simulink model "Final_hand_model"  (R2020b)
settings: Solver=VariableStepAuto  StartTime=0.0  StopTime=10.0  RelTol=1e-3  AbsTol=1e-3  EnableMultiTasking=on
values from neighbouring files (symbols this model uses):
  Out = 0    [Gesture_code_to_use_network_Arduino.m]    (also in Gesture_code_to_use_network_Both.m; Gesture_code_to_use_network_Simulink.m)
undefined symbols (not defined in the file or in its folder): X, Y, Z
libraries: sm_lib x78, nesl_utility x16
(part 1 of 3)
settings Model: Creator=Joshu  LastModifiedBy=Joshu
settings SolverCC: AutoScaleAbsTol=off
settings DataIOCC: LimitDataPoints=on  MaxDataPoints=10000
settings OptimizationCC: LifeSpan=inf
settings DebuggingCC: AllowSymbolicDim=off  SFUnexpectedBacktrackingDiag=warning  SFNoUnconditionalDefaultTransitionDiag=warning  SFExecutionAtInitializationDiag=none  ArithmeticOperatorsInVariantConditions=warning
settings SFSimCC: SimUseLocalCustomCode=off  CustomCodeUndefinedFunction=UseInterfaceOnly
settings RTWCC: RTWUseLocalCustomCode=off
settings CodeAppCC: StateflowObjectComments=on
settings GRTTargetCC: TargetLangStandard=C89/C90 (ANSI)
settings ConfigComp: CovMetricSettings=dw  CovSaveCumulativeToWorkspaceVar=on  CovSaveSingleToWorkspaceVar=on  CovExternalEMLEnable=off  CovSFcnEnable=off
settings SimscapeCC: SimscapeLogType=all  SimscapeLogSimulationStatistics=on  SimscapeLogDataHistory=10000

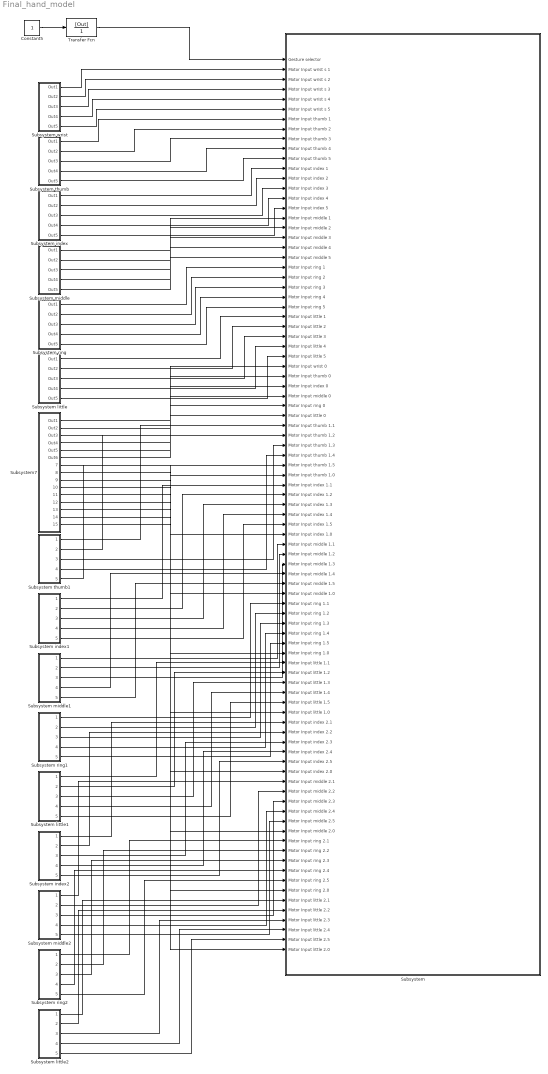
== system Final_hand_model ==
  Constant5 : Constant
  Subsystem : Subsystem
  Subsystem index : Subsystem
  Subsystem index1 : Subsystem
  Subsystem index2 : Subsystem
  Subsystem little : Subsystem
  Subsystem little1 : Subsystem
  Subsystem little2 : Subsystem
  Subsystem middle : Subsystem
  Subsystem middle1 : Subsystem
  Subsystem middle2 : Subsystem
  Subsystem ring : Subsystem
  Subsystem ring1 : Subsystem
  Subsystem ring2 : Subsystem
  Subsystem thumb : Subsystem
  Subsystem thumb1 : Subsystem
  Subsystem wrist : Subsystem
  Subsystem7 : Subsystem
  Transfer Fcn : TransferFcn  Numerator=[Out]  Denominator=[1]
  wires:
  Transfer Fcn/1 -> Subsystem/1(Gesture selector)
  Constant5/1 -> Transfer Fcn/1
  Subsystem wrist/1(Out1) -> Subsystem/2(Motor Input wrist s 1)
  Subsystem wrist/2(Out2) -> Subsystem/3(Motor Input wrist s 2)
  Subsystem wrist/3(Out3) -> Subsystem/4(Motor Input wrist s 3)
  Subsystem wrist/4(Out4) -> Subsystem/5(Motor Input wrist s 4)
  Subsystem wrist/5(Out5) -> Subsystem/6(Motor Input wrist s 5)
  Subsystem thumb/1(Out1) -> Subsystem/7(Motor Input thumb 1)
  Subsystem thumb/2(Out2) -> Subsystem/8(Motor Input thumb 2)
  Subsystem thumb/3(Out3) -> Subsystem/9(Motor Input thumb 3)
  Subsystem thumb/4(Out4) -> Subsystem/10(Motor Input thumb 4)
  Subsystem thumb/5(Out5) -> Subsystem/11(Motor Input thumb 5)
  Subsystem index/1(Out1) -> Subsystem/12(Motor Input index 1)
  Subsystem index/2(Out2) -> Subsystem/13(Motor Input index 2)
  Subsystem index/3(Out3) -> Subsystem/14(Motor Input index 3)
  Subsystem index/4(Out4) -> Subsystem/15(Motor Input index 4)
  Subsystem index/5(Out5) -> Subsystem/16(Motor Input index 5)
  Subsystem middle/1(Out1) -> Subsystem/17(Motor Input middle 1)
  Subsystem middle/2(Out2) -> Subsystem/18(Motor Input middle 2)
  Subsystem middle/3(Out3) -> Subsystem/19(Motor Input middle 3)
  Subsystem middle/4(Out4) -> Subsystem/20(Motor Input middle 4)
  Subsystem middle/5(Out5) -> Subsystem/21(Motor Input middle 5)
  Subsystem ring/1(Out1) -> Subsystem/22(Motor Input ring 1)
  Subsystem ring/2(Out2) -> Subsystem/23(Motor Input ring 2)
  Subsystem ring/3(Out3) -> Subsystem/24(Motor Input ring 3)
  Subsystem ring/4(Out4) -> Subsystem/25(Motor Input ring 4)
  Subsystem ring/5(Out5) -> Subsystem/26(Motor Input ring 5)
  Subsystem little/1(Out1) -> Subsystem/27(Motor Input little 1)
  Subsystem little/2(Out2) -> Subsystem/28(Motor Input little 2)
  Subsystem little/3(Out3) -> Subsystem/29(Motor Input little 3)
  Subsystem little/4(Out4) -> Subsystem/30(Motor Input little 4)
  Subsystem little/5(Out5) -> Subsystem/31(Motor Input little 5)
  Subsystem7/1(Out1) -> Subsystem/32(Motor Input wrist 0)
  Subsystem7/2(Out2) -> Subsystem/33(Motor Input thumb 0)
  Subsystem7/3(Out3) -> Subsystem/34(Motor Input index 0)
  Subsystem7/4(Out4) -> Subsystem/35(Motor Input middle 0)
  Subsystem7/5(Out5) -> Subsystem/36(Motor Input ring 0)
  Subsystem7/6(Out6) -> Subsystem/37(Motor Input little 0)
  Subsystem7/7(Motor Input thumb 1.0) -> Subsystem/43(Motor Input thumb 1.0)
  Subsystem7/8(Motor Input index 1.0) -> Subsystem/49(Motor Input index 1.0)
  Subsystem7/9(Motor Input middle 1.0) -> Subsystem/55(Motor Input middle 1.0)
  Subsystem7/10(Motor Input ring 1.0) -> Subsystem/61(Motor Input ring 1.0)
  Subsystem7/11(Motor Input little 1.0) -> Subsystem/67(Motor Input little 1.0)
  Subsystem7/12(Motor Input index 2.0) -> Subsystem/73(Motor Input index 2.0)
  Subsystem7/13(Motor Input middle 2.0) -> Subsystem/79(Motor Input middle 2.0)
  Subsystem7/14(Motor Input ring 2.0) -> Subsystem/85(Motor Input ring 2.0)
  Subsystem7/15(Motor Input little 2.0) -> Subsystem/91(Motor Input little 2.0)
  Subsystem thumb1/1(Motor Input thumb 1.1) -> Subsystem/38(Motor Input thumb 1.1)
  Subsystem thumb1/2(Motor Input thumb 1.2) -> Subsystem/39(Motor Input thumb 1.2)
  Subsystem thumb1/3(Motor Input thumb 1.3) -> Subsystem/40(Motor Input thumb 1.3)
  Subsystem thumb1/4(Motor Input thumb 1.4) -> Subsystem/41(Motor Input thumb 1.4)
  Subsystem thumb1/5(Motor Input thumb 1.5) -> Subsystem/42(Motor Input thumb 1.5)
  Subsystem index1/1(Motor Input index 1.1) -> Subsystem/44(Motor Input index 1.1)
  Subsystem index1/2(Motor Input index 1.2) -> Subsystem/45(Motor Input index 1.2)
  Subsystem index1/3(Motor Input index 1.3) -> Subsystem/46(Motor Input index 1.3)
  Subsystem index1/4(Motor Input index 1.4) -> Subsystem/47(Motor Input index 1.4)
  Subsystem index1/5(Motor Input index 1.5) -> Subsystem/48(Motor Input index 1.5)
  Subsystem middle1/1(Motor Input middle 1.1) -> Subsystem/50(Motor Input middle 1.1)
  Subsystem middle1/2(Motor Input middle 1.2) -> Subsystem/51(Motor Input middle 1.2)
  Subsystem middle1/3(Motor Input middle 1.3) -> Subsystem/52(Motor Input middle 1.3)
  Subsystem middle1/4(Motor Input middle 1.4) -> Subsystem/53(Motor Input middle 1.4)
  Subsystem middle1/5(Motor Input middle 1.5) -> Subsystem/54(Motor Input middle 1.5)
  Subsystem ring1/1(Motor Input ring 1.1) -> Subsystem/56(Motor Input ring 1.1)
  Subsystem ring1/2(Motor Input ring 1.2) -> Subsystem/57(Motor Input ring 1.2)
  Subsystem ring1/3(Motor Input ring 1.3) -> Subsystem/58(Motor Input ring 1.3)
  Subsystem ring1/4(Motor Input ring 1.4) -> Subsystem/59(Motor Input ring 1.4)
  Subsystem ring1/5(Motor Input ring 1.5) -> Subsystem/60(Motor Input ring 1.5)
  Subsystem little1/1(Motor Input little 1.1) -> Subsystem/62(Motor Input little 1.1)
  Subsystem little1/2(Motor Input little 1.2) -> Subsystem/63(Motor Input little 1.2)
  Subsystem little1/3(Motor Input little 1.3) -> Subsystem/64(Motor Input little 1.3)
  Subsystem little1/4(Motor Input little 1.4) -> Subsystem/65(Motor Input little 1.4)
  Subsystem little1/5(Motor Input little 1.5) -> Subsystem/66(Motor Input little 1.5)
  Subsystem index2/1(Motor Input index 2.1) -> Subsystem/68(Motor Input index 2.1)
  Subsystem index2/2(Motor Input index 2.2) -> Subsystem/69(Motor Input index 2.2)
  Subsystem index2/3(Motor Input index 2.3) -> Subsystem/70(Motor Input index 2.3)
  Subsystem index2/4(Motor Input index 2.4) -> Subsystem/71(Motor Input index 2.4)
  Subsystem index2/5(Motor Input index 2.5) -> Subsystem/72(Motor Input index 2.5)
  Subsystem middle2/1(Motor Input middle 2.1) -> Subsystem/74(Motor Input middle 2.1)
  Subsystem middle2/2(Motor Input middle 2.2) -> Subsystem/75(Motor Input middle 2.2)
  Subsystem middle2/3(Motor Input middle 2.3) -> Subsystem/76(Motor Input middle 2.3)
  Subsystem middle2/4(Motor Input middle 2.4) -> Subsystem/77(Motor Input middle 2.4)
  Subsystem middle2/5(Motor Input middle 2.5) -> Subsystem/78(Motor Input middle 2.5)
  Subsystem ring2/1(Motor Input ring 2.1) -> Subsystem/80(Motor Input ring 2.1)
  Subsystem ring2/2(Motor Input ring 2.2) -> Subsystem/81(Motor Input ring 2.2)
  Subsystem ring2/3(Motor Input ring 2.3) -> Subsystem/82(Motor Input ring 2.3)
  Subsystem ring2/4(Motor Input ring 2.4) -> Subsystem/83(Motor Input ring 2.4)
  Subsystem ring2/5(Motor Input ring 2.5) -> Subsystem/84(Motor Input ring 2.5)
  Subsystem little2/1(Motor Input little 2.1) -> Subsystem/86(Motor Input little 2.1)
  Subsystem little2/2(Motor Input little 2.2) -> Subsystem/87(Motor Input little 2.2)
  Subsystem little2/3(Motor Input little 2.3) -> Subsystem/88(Motor Input little 2.3)
  Subsystem little2/4(Motor Input little 2.4) -> Subsystem/89(Motor Input little 2.4)
  Subsystem little2/5(Motor Input little 2.5) -> Subsystem/90(Motor Input little 2.5)

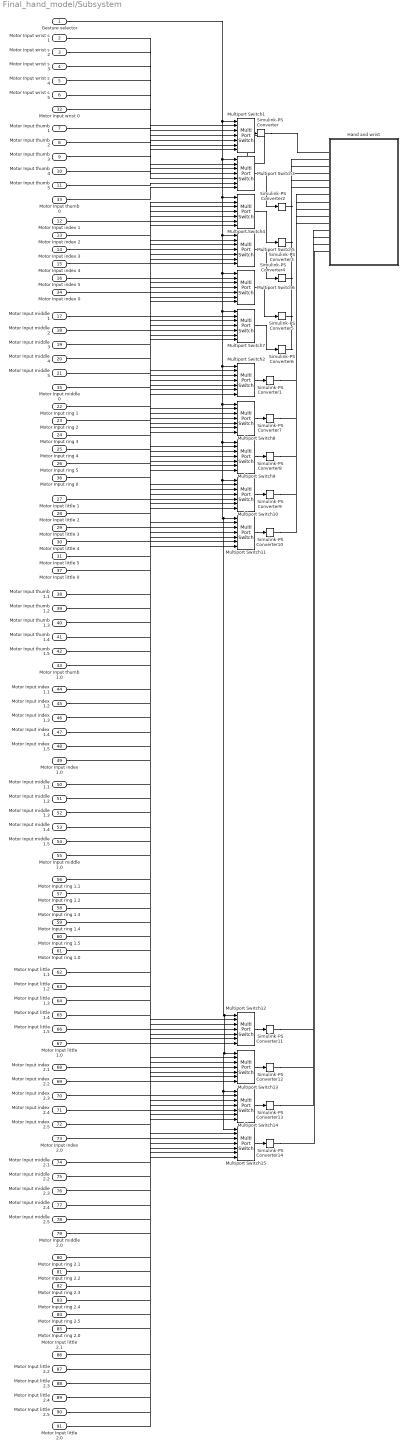
== system Final_hand_model/Subsystem ==
  Gesture selector : Inport
  Motor Input wrist s 1 : Inport  Port=2
  Motor Input wrist s 2 : Inport  Port=3
  Motor Input wrist s 3 : Inport  Port=4
  Motor Input wrist s 4 : Inport  Port=5
  Motor Input wrist s 5 : Inport  Port=6
  Motor Input thumb 1 : Inport  Port=7
  Motor Input thumb 2 : Inport  Port=8
  Motor Input thumb 3 : Inport  Port=9
  Motor Input thumb 4 : Inport  Port=10
  Motor Input thumb 5 : Inport  Port=11
  Motor Input index 1 : Inport  Port=12
  Motor Input index 2 : Inport  Port=13
  Motor Input index 3 : Inport  Port=14
  Motor Input index 4 : Inport  Port=15
  Motor Input index 5 : Inport  Port=16
  Motor Input middle 1 : Inport  Port=17
  Motor Input middle 2 : Inport  Port=18
  Motor Input middle 3 : Inport  Port=19
  Motor Input middle 4 : Inport  Port=20
  Motor Input middle 5 : Inport  Port=21
  Motor Input ring 1 : Inport  Port=22
  Motor Input ring 2 : Inport  Port=23
  Motor Input ring 3 : Inport  Port=24
  Motor Input ring 4 : Inport  Port=25
  Motor Input ring 5 : Inport  Port=26
  Motor Input little 1 : Inport  Port=27
  Motor Input little 2 : Inport  Port=28
  Motor Input little 3 : Inport  Port=29
  Motor Input little 4 : Inport  Port=30
  Motor Input little 5 : Inport  Port=31
  Motor Input wrist 0 : Inport  Port=32
  Motor Input thumb 0 : Inport  Port=33
  Motor Input index 0 : Inport  Port=34
  Motor Input middle 0 : Inport  Port=35
  Motor Input ring 0 : Inport  Port=36
  Motor Input little 0 : Inport  Port=37
  Motor Input thumb 1.1 : Inport  Port=38
  Motor Input thumb 1.2 : Inport  Port=39
  Motor Input thumb 1.3 : Inport  Port=40
  Motor Input thumb 1.4 : Inport  Port=41
  Motor Input thumb 1.5 : Inport  Port=42
  Motor Input thumb 1.0 : Inport  Port=43
  Motor Input index 1.1 : Inport  Port=44
  Motor Input index 1.2 : Inport  Port=45
  Motor Input index 1.3 : Inport  Port=46
  Motor Input index 1.4 : Inport  Port=47
  Motor Input index 1.5 : Inport  Port=48
  Motor Input index 1.0 : Inport  Port=49
  Motor Input middle 1.1 : Inport  Port=50
  Motor Input middle 1.2 : Inport  Port=51
  Motor Input middle 1.3 : Inport  Port=52
  Motor Input middle 1.4 : Inport  Port=53
  Motor Input middle 1.5 : Inport  Port=54
  Motor Input middle 1.0 : Inport  Port=55
  Motor Input ring 1.1 : Inport  Port=56
  Motor Input ring 1.2 : Inport  Port=57
  Motor Input ring 1.3 : Inport  Port=58
  Motor Input ring 1.4 : Inport  Port=59
  Motor Input ring 1.5 : Inport  Port=60
  Motor Input ring 1.0 : Inport  Port=61
  Motor Input little 1.1 : Inport  Port=62
  Motor Input little 1.2 : Inport  Port=63
  Motor Input little 1.3 : Inport  Port=64
  Motor Input little 1.4 : Inport  Port=65
  Motor Input little 1.5 : Inport  Port=66
  Motor Input little 1.0 : Inport  Port=67
  Motor Input index 2.1 : Inport  Port=68
  Motor Input index 2.2 : Inport  Port=69
  Motor Input index 2.3 : Inport  Port=70
  Motor Input index 2.4 : Inport  Port=71
  Motor Input index 2.5 : Inport  Port=72
  Motor Input index 2.0 : Inport  Port=73
  Motor Input middle 2.1 : Inport  Port=74
  Motor Input middle 2.2 : Inport  Port=75
  Motor Input middle 2.3 : Inport  Port=76
  Motor Input middle 2.4 : Inport  Port=77
  Motor Input middle 2.5 : Inport  Port=78
  Motor Input middle 2.0 : Inport  Port=79
  Motor Input ring 2.1 : Inport  Port=80
  Motor Input ring 2.2 : Inport  Port=81
  Motor Input ring 2.3 : Inport  Port=82
  Motor Input ring 2.4 : Inport  Port=83
  Motor Input ring 2.5 : Inport  Port=84
  Motor Input ring 2.0 : Inport  Port=85
  Motor Input little 2.1 : Inport  Port=86
  Motor Input little 2.2 : Inport  Port=87
  Motor Input little 2.3 : Inport  Port=88
  Motor Input little 2.4 : Inport  Port=89
  Motor Input little 2.5 : Inport  Port=90
  Motor Input little 2.0 : Inport  Port=91
  Hand and wrist : Subsystem
  Multiport Switch{1..15} (15 alike) : MultiPortSwitch  Inputs=5  DataPortForDefault=Additional data port  DiagnosticForDefault=None
  Simulink-PS Converter{,1..14} (15 alike) : nesl_utility/Simulink-PS Converter  PhysicalDomain=network_engine_domain  SubClassName=ps_input  LeftPortType=input  RightPortType=output  PseudoPeriodic=off  Frequencies=[]  NoiseDistribution=none  NoiseParameters=[]  Unit=1  AffineConversion=off  FilteringAndDerivatives=filter  SimscapeFilterOrder=2  InputFilterTimeConstant=0.001  UdotUserProvided=0
  wires:
  Motor Input ring 3/1 -> Multiport Switch6/4
  Motor Input thumb 2/1 -> Multiport Switch3/3
  Multiport Switch1/1 -> Simulink-PS Converter/1
  Motor Input wrist s 4/1 -> Multiport Switch1/5
  Motor Input index 1/1 -> Multiport Switch4/2
  Motor Input thumb 3/1 -> Multiport Switch3/4
  Motor Input little 1/1 -> Multiport Switch7/2
  Multiport Switch4/1 -> Simulink-PS Converter3/1
  Multiport Switch5/1 -> Simulink-PS Converter4/1
  Multiport Switch6/1 -> Simulink-PS Converter5/1
  Motor Input wrist s 5/1 -> Multiport Switch1/6
  Motor Input middle 1/1 -> Multiport Switch5/2
  Motor Input little 3/1 -> Multiport Switch7/4
  Motor Input ring 5/1 -> Multiport Switch6/6
  Motor Input thumb 5/1 -> Multiport Switch3/6
  Motor Input thumb 1/1 -> Multiport Switch3/2
  Motor Input middle 5/1 -> Multiport Switch5/6
  Motor Input index 3/1 -> Multiport Switch4/4
  Motor Input wrist s 3/1 -> Multiport Switch1/4
  Motor Input little 4/1 -> Multiport Switch7/5
  Multiport Switch3/1 -> Simulink-PS Converter2/1
  Motor Input wrist s 2/1 -> Multiport Switch1/3
  Motor Input little 2/1 -> Multiport Switch7/3
  Motor Input index 5/1 -> Multiport Switch4/6
  Motor Input ring 2/1 -> Multiport Switch6/3
  Motor Input middle 4/1 -> Multiport Switch5/5
  Motor Input index 2/1 -> Multiport Switch4/3
  Motor Input ring 1/1 -> Multiport Switch6/2
  Gesture selector/1 -> Multiport Switch2/1, Multiport Switch12/1, Multiport Switch15/1, Multiport Switch14/1, Multiport Switch13/1, Multiport Switch11/1, Multiport Switch10/1, Multiport Switch9/1, Multiport Switch8/1, Multiport Switch7/1, Multiport Switch6/1, Multiport Switch5/1, Multiport Switch4/1, Multiport Switch3/1, Multiport Switch1/1
  Multiport Switch7/1 -> Simulink-PS Converter6/1
  Motor Input thumb 4/1 -> Multiport Switch3/5
  Motor Input ring 4/1 -> Multiport Switch6/5
  Motor Input middle 3/1 -> Multiport Switch5/4
  Motor Input middle 2/1 -> Multiport Switch5/3
  Motor Input index 4/1 -> Multiport Switch4/5
  Motor Input wrist s 1/1 -> Multiport Switch1/2
  Motor Input little 5/1 -> Multiport Switch7/6
  Motor Input wrist 0/1 -> Multiport Switch1/7
  Motor Input thumb 0/1 -> Multiport Switch3/7
  Motor Input index 0/1 -> Multiport Switch4/7
  Motor Input middle 0/1 -> Multiport Switch5/7
  Motor Input ring 0/1 -> Multiport Switch6/7
  Motor Input little 0/1 -> Multiport Switch7/7
  Multiport Switch2/1 -> Simulink-PS Converter1/1
  Multiport Switch8/1 -> Simulink-PS Converter7/1
  Multiport Switch9/1 -> Simulink-PS Converter8/1
  Multiport Switch10/1 -> Simulink-PS Converter9/1
  Multiport Switch11/1 -> Simulink-PS Converter10/1
  Multiport Switch12/1 -> Simulink-PS Converter11/1
  Multiport Switch13/1 -> Simulink-PS Converter12/1
  Multiport Switch14/1 -> Simulink-PS Converter13/1
  Multiport Switch15/1 -> Simulink-PS Converter14/1
  Motor Input thumb 1.1/1 -> Multiport Switch2/2
  Motor Input thumb 1.2/1 -> Multiport Switch2/3
  Motor Input thumb 1.3/1 -> Multiport Switch2/4
  Motor Input thumb 1.4/1 -> Multiport Switch2/5
  Motor Input thumb 1.5/1 -> Multiport Switch2/6
  Motor Input thumb 1.0/1 -> Multiport Switch2/7
  Motor Input index 1.1/1 -> Multiport Switch8/2
  Motor Input index 1.2/1 -> Multiport Switch8/3
  Motor Input index 1.3/1 -> Multiport Switch8/4
  Motor Input index 1.4/1 -> Multiport Switch8/5
  Motor Input index 1.5/1 -> Multiport Switch8/6
  Motor Input index 1.0/1 -> Multiport Switch8/7
  Motor Input middle 1.1/1 -> Multiport Switch9/2
  Motor Input middle 1.2/1 -> Multiport Switch9/3
  Motor Input middle 1.3/1 -> Multiport Switch9/4
  Motor Input middle 1.4/1 -> Multiport Switch9/5
  Motor Input middle 1.5/1 -> Multiport Switch9/6
  Motor Input middle 1.0/1 -> Multiport Switch9/7
  Motor Input ring 1.1/1 -> Multiport Switch10/2
  Motor Input ring 1.2/1 -> Multiport Switch10/3
  Motor Input ring 1.3/1 -> Multiport Switch10/4
  Motor Input ring 1.4/1 -> Multiport Switch10/5
  Motor Input ring 1.5/1 -> Multiport Switch10/6
  Motor Input ring 1.0/1 -> Multiport Switch10/7
  Motor Input little 1.1/1 -> Multiport Switch11/2
  Motor Input little 1.2/1 -> Multiport Switch11/3
  Motor Input little 1.3/1 -> Multiport Switch11/4
  Motor Input little 1.4/1 -> Multiport Switch11/5
  Motor Input little 1.5/1 -> Multiport Switch11/6
  Motor Input little 1.0/1 -> Multiport Switch11/7
  Motor Input index 2.1/1 -> Multiport Switch12/2
  Motor Input index 2.2/1 -> Multiport Switch12/3
  Motor Input index 2.3/1 -> Multiport Switch12/4
  Motor Input index 2.4/1 -> Multiport Switch12/5
  Motor Input index 2.5/1 -> Multiport Switch12/6
  Motor Input index 2.0/1 -> Multiport Switch12/7
  Motor Input middle 2.1/1 -> Multiport Switch13/2
  Motor Input middle 2.2/1 -> Multiport Switch13/3
  Motor Input middle 2.3/1 -> Multiport Switch13/4
  Motor Input middle 2.4/1 -> Multiport Switch13/5
  Motor Input middle 2.5/1 -> Multiport Switch13/6
  Motor Input middle 2.0/1 -> Multiport Switch13/7
  Motor Input ring 2.1/1 -> Multiport Switch14/2
  Motor Input ring 2.2/1 -> Multiport Switch14/3
  Motor Input ring 2.3/1 -> Multiport Switch14/4
  Motor Input ring 2.4/1 -> Multiport Switch14/5
  Motor Input ring 2.5/1 -> Multiport Switch14/6
  Motor Input ring 2.0/1 -> Multiport Switch14/7
  Motor Input little 2.1/1 -> Multiport Switch15/2
  Motor Input little 2.2/1 -> Multiport Switch15/3
  Motor Input little 2.3/1 -> Multiport Switch15/4
  Motor Input little 2.4/1 -> Multiport Switch15/5
  Motor Input little 2.5/1 -> Multiport Switch15/6
  Motor Input little 2.0/1 -> Multiport Switch15/7
  connections:
  Simulink-PS Converter/RConn1 -- Hand and wrist/RConn1
  Simulink-PS Converter3/RConn1 -- Hand and wrist/RConn3
  Simulink-PS Converter2/RConn1 -- Hand and wrist/RConn2
  Simulink-PS Converter4/RConn1 -- Hand and wrist/RConn4
  Simulink-PS Converter6/RConn1 -- Hand and wrist/RConn6
  Simulink-PS Converter5/RConn1 -- Hand and wrist/RConn5
  Simulink-PS Converter1/RConn1 -- Hand and wrist/RConn7
  Simulink-PS Converter7/RConn1 -- Hand and wrist/RConn8
  Simulink-PS Converter8/RConn1 -- Hand and wrist/RConn9
  Simulink-PS Converter9/RConn1 -- Hand and wrist/RConn10
  Simulink-PS Converter10/RConn1 -- Hand and wrist/RConn11
  Simulink-PS Converter11/RConn1 -- Hand and wrist/RConn12
  Simulink-PS Converter12/RConn1 -- Hand and wrist/RConn13
  Simulink-PS Converter13/RConn1 -- Hand and wrist/RConn14
  Simulink-PS Converter14/RConn1 -- Hand and wrist/RConn15

== system Final_hand_model/Subsystem index ==
  " scissors index" : Constant  Value=0
  Constant16 : Constant  Value=0
  Dead Zone1 : DeadZone  LowerValue=-10  UpperValue=0  SaturateOnIntegerOverflow=on
  Dead Zone2 : DeadZone  LowerValue=-10  UpperValue=0  SaturateOnIntegerOverflow=on
  Dead Zone3 : DeadZone  LowerValue=-10  UpperValue=0  SaturateOnIntegerOverflow=on
  Sine Wave Balala index : Sin  Amplitude=0.5  Frequency=3  Phase=3*pi/5  SampleTime=0
  Sine Wave Fist index : Sin  Amplitude=1.3  Frequency=3  SampleTime=0
  Sine Wave swear index : Sin  Amplitude=1.3  Frequency=3  SampleTime=0
  Out1 : Outport
  Out2 : Outport  Port=2
  Out3 : Outport  Port=3
  Out4 : Outport  Port=4
  Out5 : Outport  Port=5
  wires:
  Sine Wave Fist index/1 -> Dead Zone2/1
  " scissors index"/1 -> Out4/1
  Dead Zone2/1 -> Out1/1
  Dead Zone1/1 -> Out5/1
  Dead Zone3/1 -> Out3/1
  Constant16/1 -> Out2/1
  Sine Wave Balala index/1 -> Dead Zone3/1
  Sine Wave swear index/1 -> Dead Zone1/1

== system Final_hand_model/Subsystem index1 ==
  " scissors index" : Constant  Value=0
  Constant16 : Constant  Value=0
  Dead Zone1 : DeadZone  LowerValue=-10  UpperValue=0  SaturateOnIntegerOverflow=on
  Dead Zone2 : DeadZone  LowerValue=-10  UpperValue=0  SaturateOnIntegerOverflow=on
  Dead Zone3 : DeadZone  LowerValue=-10  UpperValue=0  SaturateOnIntegerOverflow=on
  Sine Wave Balala index : Sin  Amplitude=0.5  Frequency=3  Phase=3*pi/5  SampleTime=0
  Sine Wave Fist index : Sin  Amplitude=1.3  Frequency=3  SampleTime=0
  Sine Wave swear index : Sin  Amplitude=1.3  Frequency=3  SampleTime=0
  Motor Input index 1.1 : Outport
  Motor Input index 1.2 : Outport  Port=2
  Motor Input index 1.3 : Outport  Port=3
  Motor Input index 1.4 : Outport  Port=4
  Motor Input index 1.5 : Outport  Port=5
  wires:
  Sine Wave Fist index/1 -> Dead Zone2/1
  " scissors index"/1 -> Motor Input index 1.4/1
  Dead Zone2/1 -> Motor Input index 1.1/1
  Dead Zone1/1 -> Motor Input index 1.5/1
  Dead Zone3/1 -> Motor Input index 1.3/1
  Constant16/1 -> Motor Input index 1.2/1
  Sine Wave Balala index/1 -> Dead Zone3/1
  Sine Wave swear index/1 -> Dead Zone1/1

== system Final_hand_model/Subsystem index2 ==
  " scissors index" : Constant  Value=0
  Constant16 : Constant  Value=0
  Dead Zone1 : DeadZone  LowerValue=-10  UpperValue=0  SaturateOnIntegerOverflow=on
  Dead Zone2 : DeadZone  LowerValue=-10  UpperValue=0  SaturateOnIntegerOverflow=on
  Dead Zone3 : DeadZone  LowerValue=-10  UpperValue=0  SaturateOnIntegerOverflow=on
  Sine Wave Balala index : Sin  Amplitude=0.5  Frequency=3  Phase=3*pi/5  SampleTime=0
  Sine Wave Fist index : Sin  Amplitude=1.3  Frequency=3  SampleTime=0
  Sine Wave swear index : Sin  Amplitude=1.3  Frequency=3  SampleTime=0
  Motor Input index 2.1 : Outport
  Motor Input index 2.2 : Outport  Port=2
  Motor Input index 2.3 : Outport  Port=3
  Motor Input index 2.4 : Outport  Port=4
  Motor Input index 2.5 : Outport  Port=5
  wires:
  Sine Wave Fist index/1 -> Dead Zone2/1
  " scissors index"/1 -> Motor Input index 2.4/1
  Dead Zone2/1 -> Motor Input index 2.1/1
  Dead Zone1/1 -> Motor Input index 2.5/1
  Dead Zone3/1 -> Motor Input index 2.3/1
  Constant16/1 -> Motor Input index 2.2/1
  Sine Wave Balala index/1 -> Dead Zone3/1
  Sine Wave swear index/1 -> Dead Zone1/1

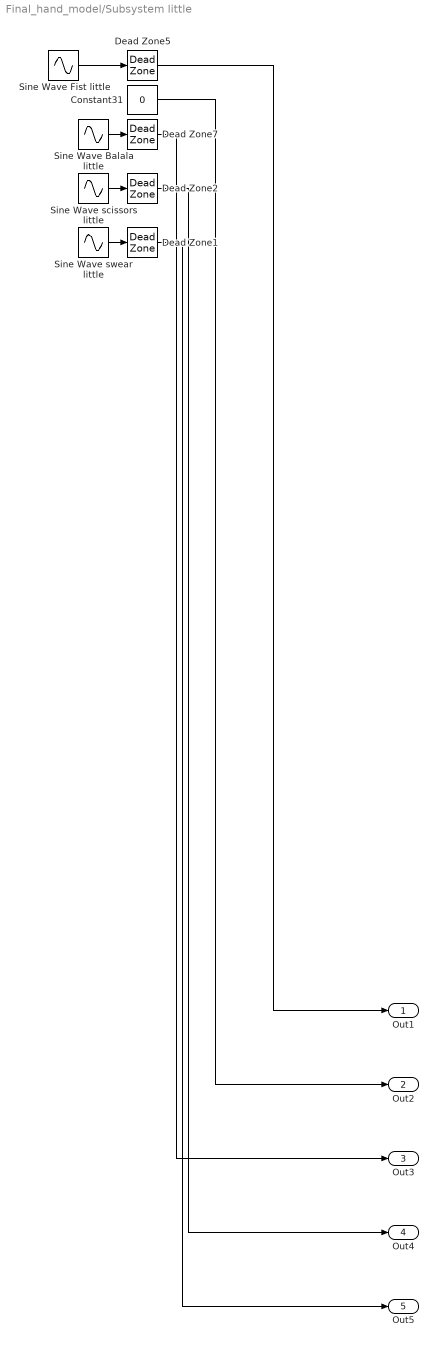
== system Final_hand_model/Subsystem little ==
  Constant31 : Constant  Value=0
  Dead Zone{1..2,5,7} (4 alike) : DeadZone  LowerValue=-10  UpperValue=0  SaturateOnIntegerOverflow=on
  Sine Wave Balala little : Sin  Amplitude=0.5  Frequency=3  SampleTime=0
  Sine Wave Fist little : Sin  Amplitude=1.3  Frequency=3  SampleTime=0
  Sine Wave scissors little : Sin  Amplitude=1.3  Frequency=3  SampleTime=0
  Sine Wave swear little : Sin  Amplitude=1.3  Frequency=3  SampleTime=0
  Out1 : Outport
  Out2 : Outport  Port=2
  Out3 : Outport  Port=3
  Out4 : Outport  Port=4
  Out5 : Outport  Port=5
  wires:
  Sine Wave Fist little/1 -> Dead Zone5/1
  Dead Zone1/1 -> Out5/1
  Dead Zone7/1 -> Out3/1
  Constant31/1 -> Out2/1
  Dead Zone2/1 -> Out4/1
  Dead Zone5/1 -> Out1/1
  Sine Wave Balala little/1 -> Dead Zone7/1
  Sine Wave scissors little/1 -> Dead Zone2/1
  Sine Wave swear little/1 -> Dead Zone1/1

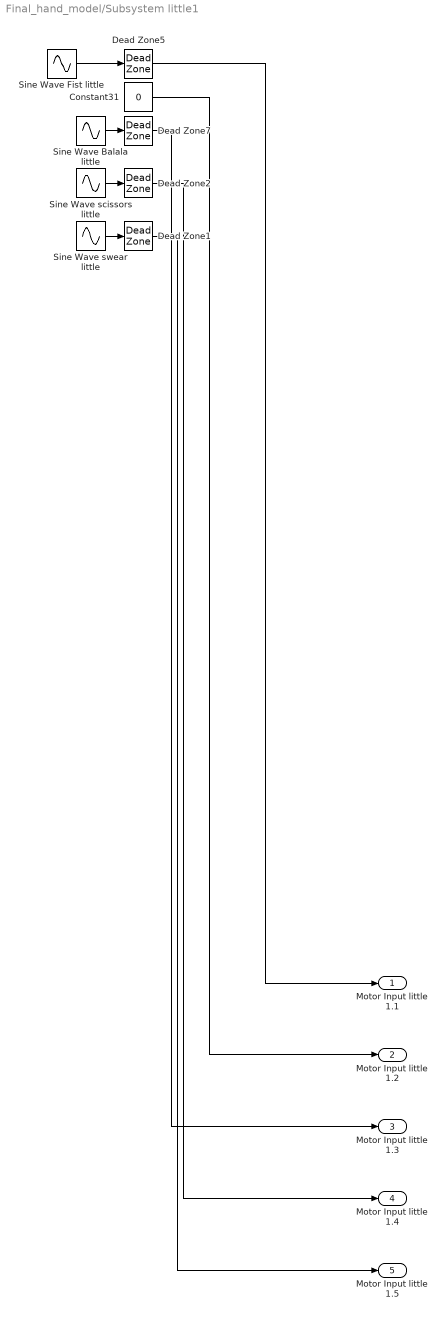
== system Final_hand_model/Subsystem little1 ==
  Constant31 : Constant  Value=0
  Dead Zone{1..2,5,7} (4 alike) : DeadZone  LowerValue=-10  UpperValue=0  SaturateOnIntegerOverflow=on
  Sine Wave Balala little : Sin  Amplitude=0.5  Frequency=3  SampleTime=0
  Sine Wave Fist little : Sin  Amplitude=1.3  Frequency=3  SampleTime=0
  Sine Wave scissors little : Sin  Amplitude=1.3  Frequency=3  SampleTime=0
  Sine Wave swear little : Sin  Amplitude=1.3  Frequency=3  SampleTime=0
  Motor Input little 1.1 : Outport
  Motor Input little 1.2 : Outport  Port=2
  Motor Input little 1.3 : Outport  Port=3
  Motor Input little 1.4 : Outport  Port=4
  Motor Input little 1.5 : Outport  Port=5
  wires:
  Sine Wave Fist little/1 -> Dead Zone5/1
  Dead Zone1/1 -> Motor Input little 1.5/1
  Dead Zone7/1 -> Motor Input little 1.3/1
  Constant31/1 -> Motor Input little 1.2/1
  Dead Zone2/1 -> Motor Input little 1.4/1
  Dead Zone5/1 -> Motor Input little 1.1/1
  Sine Wave Balala little/1 -> Dead Zone7/1
  Sine Wave scissors little/1 -> Dead Zone2/1
  Sine Wave swear little/1 -> Dead Zone1/1

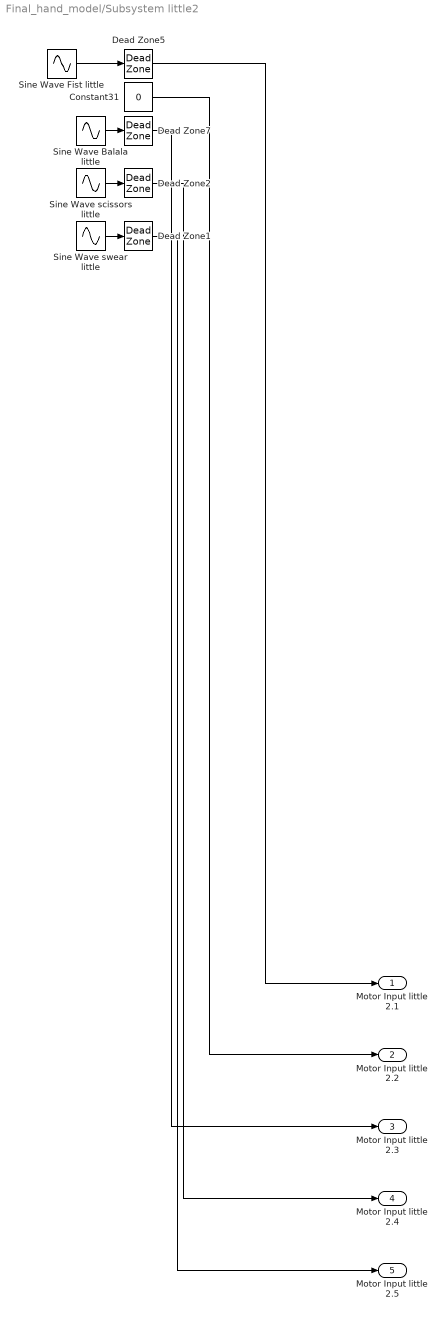
== system Final_hand_model/Subsystem little2 ==
  Constant31 : Constant  Value=0
  Dead Zone{1..2,5,7} (4 alike) : DeadZone  LowerValue=-10  UpperValue=0  SaturateOnIntegerOverflow=on
  Sine Wave Balala little : Sin  Amplitude=0.5  Frequency=3  SampleTime=0
  Sine Wave Fist little : Sin  Amplitude=1.3  Frequency=3  SampleTime=0
  Sine Wave scissors little : Sin  Amplitude=1.3  Frequency=3  SampleTime=0
  Sine Wave swear little : Sin  Amplitude=1.3  Frequency=3  SampleTime=0
  Motor Input little 2.1 : Outport
  Motor Input little 2.2 : Outport  Port=2
  Motor Input little 2.3 : Outport  Port=3
  Motor Input little 2.4 : Outport  Port=4
  Motor Input little 2.5 : Outport  Port=5
  wires:
  Sine Wave Fist little/1 -> Dead Zone5/1
  Dead Zone1/1 -> Motor Input little 2.5/1
  Dead Zone7/1 -> Motor Input little 2.3/1
  Constant31/1 -> Motor Input little 2.2/1
  Dead Zone2/1 -> Motor Input little 2.4/1
  Dead Zone5/1 -> Motor Input little 2.1/1
  Sine Wave Balala little/1 -> Dead Zone7/1
  Sine Wave scissors little/1 -> Dead Zone2/1
  Sine Wave swear little/1 -> Dead Zone1/1

== system Final_hand_model/Subsystem middle ==
  Constant21 : Constant  Value=0
  Dead Zone2 : DeadZone  LowerValue=-10  UpperValue=0  SaturateOnIntegerOverflow=on
  Dead Zone3 : DeadZone  LowerValue=-10  UpperValue=0  SaturateOnIntegerOverflow=on
  Sine Wave Balala middle : Sin  Amplitude=0.5  Frequency=3  Phase=2*pi/5  SampleTime=0
  Sine Wave Fist Middle : Sin  Amplitude=1.3  Frequency=3  SampleTime=0
  scissors Middle : Constant  Value=0
  swear Middle : Constant  Value=0
  Out1 : Outport
  Out2 : Outport  Port=2
  Out3 : Outport  Port=3
  Out4 : Outport  Port=4
  Out5 : Outport  Port=5
  wires:
  swear Middle/1 -> Out5/1
  Sine Wave Fist Middle/1 -> Dead Zone3/1
  Constant21/1 -> Out2/1
  scissors Middle/1 -> Out4/1
  Dead Zone3/1 -> Out1/1
  Dead Zone2/1 -> Out3/1
  Sine Wave Balala middle/1 -> Dead Zone2/1

== system Final_hand_model/Subsystem middle1 ==
  Constant21 : Constant  Value=0
  Dead Zone2 : DeadZone  LowerValue=-10  UpperValue=0  SaturateOnIntegerOverflow=on
  Dead Zone3 : DeadZone  LowerValue=-10  UpperValue=0  SaturateOnIntegerOverflow=on
  Sine Wave Balala middle : Sin  Amplitude=0.5  Frequency=3  Phase=2*pi/5  SampleTime=0
  Sine Wave Fist Middle : Sin  Amplitude=1.3  Frequency=3  SampleTime=0
  scissors Middle : Constant  Value=0
  swear Middle : Constant  Value=0
  Motor Input middle 1.1 : Outport
  Motor Input middle 1.2 : Outport  Port=2
  Motor Input middle 1.3 : Outport  Port=3
  Motor Input middle 1.4 : Outport  Port=4
  Motor Input middle 1.5 : Outport  Port=5
  wires:
  swear Middle/1 -> Motor Input middle 1.5/1
  Sine Wave Fist Middle/1 -> Dead Zone3/1
  Constant21/1 -> Motor Input middle 1.2/1
  scissors Middle/1 -> Motor Input middle 1.4/1
  Dead Zone3/1 -> Motor Input middle 1.1/1
  Dead Zone2/1 -> Motor Input middle 1.3/1
  Sine Wave Balala middle/1 -> Dead Zone2/1

== system Final_hand_model/Subsystem middle2 ==
  Constant21 : Constant  Value=0
  Dead Zone2 : DeadZone  LowerValue=-10  UpperValue=0  SaturateOnIntegerOverflow=on
  Dead Zone3 : DeadZone  LowerValue=-10  UpperValue=0  SaturateOnIntegerOverflow=on
  Sine Wave Balala middle : Sin  Amplitude=0.5  Frequency=3  Phase=2*pi/5  SampleTime=0
  Sine Wave Fist Middle : Sin  Amplitude=1.3  Frequency=3  SampleTime=0
  scissors Middle : Constant  Value=0
  swear Middle : Constant  Value=0
  Motor Input middle 2.1 : Outport
  Motor Input middle 2.2 : Outport  Port=2
  Motor Input middle 2.3 : Outport  Port=3
  Motor Input middle 2.4 : Outport  Port=4
  Motor Input middle 2.5 : Outport  Port=5
  wires:
  swear Middle/1 -> Motor Input middle 2.5/1
  Sine Wave Fist Middle/1 -> Dead Zone3/1
  Constant21/1 -> Motor Input middle 2.2/1
  scissors Middle/1 -> Motor Input middle 2.4/1
  Dead Zone3/1 -> Motor Input middle 2.1/1
  Dead Zone2/1 -> Motor Input middle 2.3/1
  Sine Wave Balala middle/1 -> Dead Zone2/1

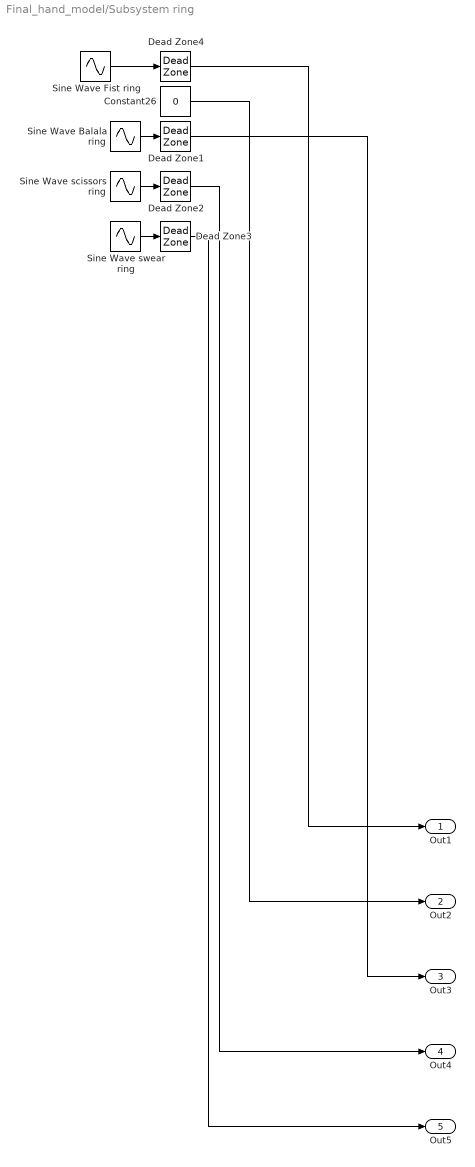
== system Final_hand_model/Subsystem ring ==
  Constant26 : Constant  Value=0
  Dead Zone{1..4} (4 alike) : DeadZone  LowerValue=-10  UpperValue=0  SaturateOnIntegerOverflow=on
  Sine Wave Balala ring : Sin  Amplitude=0.5  Frequency=3  Phase=pi/5  SampleTime=0
  Sine Wave Fist ring : Sin  Amplitude=1.3  Frequency=3  SampleTime=0
  Sine Wave scissors ring : Sin  Amplitude=1.3  Frequency=3  SampleTime=0
  Sine Wave swear ring : Sin  Amplitude=1.3  Frequency=3  SampleTime=0
  Out1 : Outport
  Out2 : Outport  Port=2
  Out3 : Outport  Port=3
  Out4 : Outport  Port=4
  Out5 : Outport  Port=5
  wires:
  Sine Wave Fist ring/1 -> Dead Zone4/1
  Dead Zone3/1 -> Out5/1
  Constant26/1 -> Out2/1
  Dead Zone2/1 -> Out4/1
  Dead Zone1/1 -> Out3/1
  Dead Zone4/1 -> Out1/1
  Sine Wave Balala ring/1 -> Dead Zone1/1
  Sine Wave scissors ring/1 -> Dead Zone2/1
  Sine Wave swear ring/1 -> Dead Zone3/1

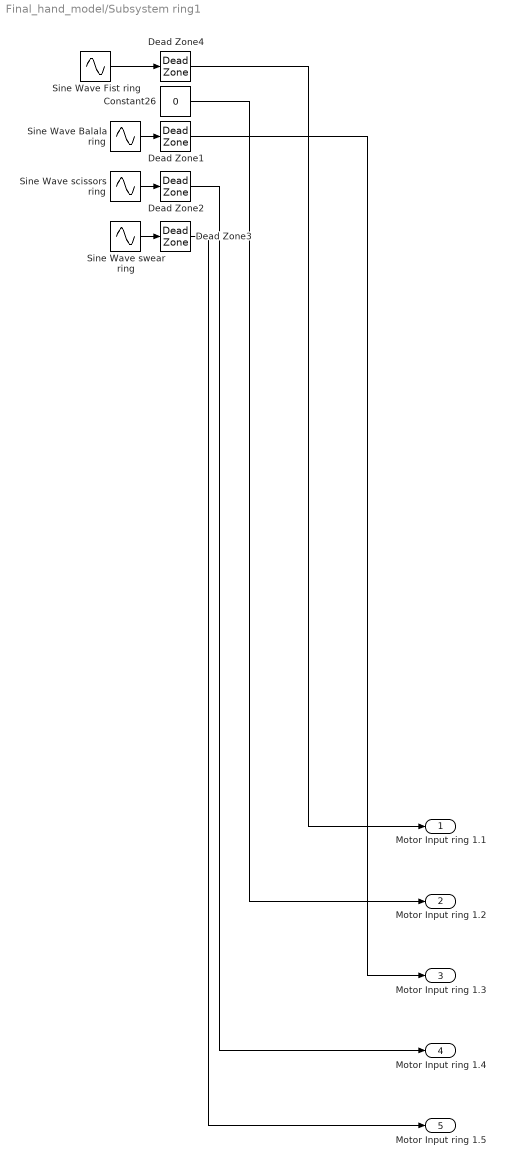
== system Final_hand_model/Subsystem ring1 ==
  Constant26 : Constant  Value=0
  Dead Zone{1..4} (4 alike) : DeadZone  LowerValue=-10  UpperValue=0  SaturateOnIntegerOverflow=on
  Sine Wave Balala ring : Sin  Amplitude=0.5  Frequency=3  Phase=pi/5  SampleTime=0
  Sine Wave Fist ring : Sin  Amplitude=1.3  Frequency=3  SampleTime=0
  Sine Wave scissors ring : Sin  Amplitude=1.3  Frequency=3  SampleTime=0
  Sine Wave swear ring : Sin  Amplitude=1.3  Frequency=3  SampleTime=0
  Motor Input ring 1.1 : Outport
  Motor Input ring 1.2 : Outport  Port=2
  Motor Input ring 1.3 : Outport  Port=3
  Motor Input ring 1.4 : Outport  Port=4
  Motor Input ring 1.5 : Outport  Port=5
  wires:
  Sine Wave Fist ring/1 -> Dead Zone4/1
  Dead Zone3/1 -> Motor Input ring 1.5/1
  Constant26/1 -> Motor Input ring 1.2/1
  Dead Zone2/1 -> Motor Input ring 1.4/1
  Dead Zone1/1 -> Motor Input ring 1.3/1
  Dead Zone4/1 -> Motor Input ring 1.1/1
  Sine Wave Balala ring/1 -> Dead Zone1/1
  Sine Wave scissors ring/1 -> Dead Zone2/1
  Sine Wave swear ring/1 -> Dead Zone3/1

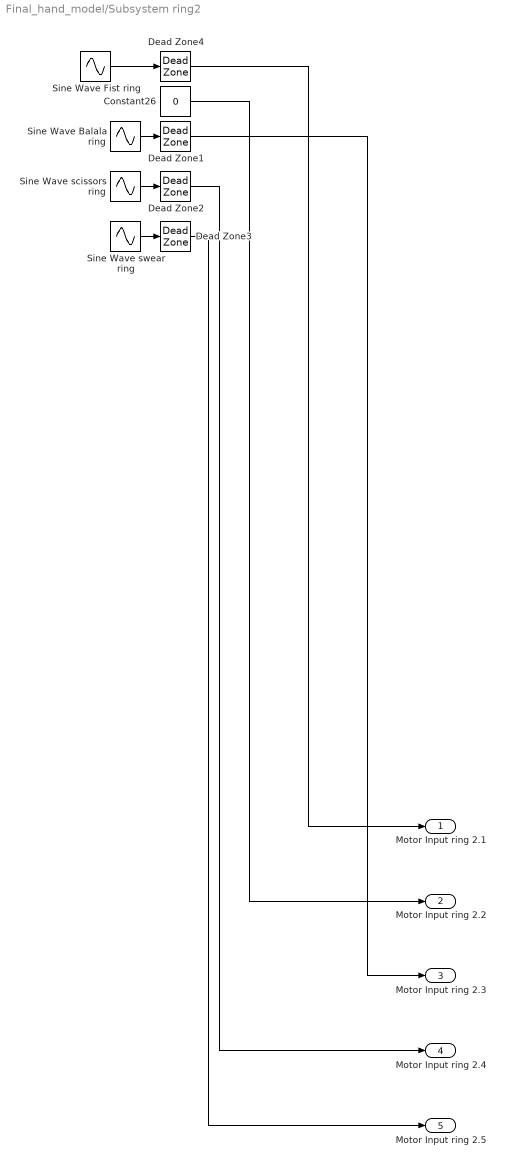
== system Final_hand_model/Subsystem ring2 ==
  Constant26 : Constant  Value=0
  Dead Zone{1..4} (4 alike) : DeadZone  LowerValue=-10  UpperValue=0  SaturateOnIntegerOverflow=on
  Sine Wave Balala ring : Sin  Amplitude=0.5  Frequency=3  Phase=pi/5  SampleTime=0
  Sine Wave Fist ring : Sin  Amplitude=1.3  Frequency=3  SampleTime=0
  Sine Wave scissors ring : Sin  Amplitude=1.3  Frequency=3  SampleTime=0
  Sine Wave swear ring : Sin  Amplitude=1.3  Frequency=3  SampleTime=0
  Motor Input ring 2.1 : Outport
  Motor Input ring 2.2 : Outport  Port=2
  Motor Input ring 2.3 : Outport  Port=3
  Motor Input ring 2.4 : Outport  Port=4
  Motor Input ring 2.5 : Outport  Port=5
  wires:
  Sine Wave Fist ring/1 -> Dead Zone4/1
  Dead Zone3/1 -> Motor Input ring 2.5/1
  Constant26/1 -> Motor Input ring 2.2/1
  Dead Zone2/1 -> Motor Input ring 2.4/1
  Dead Zone1/1 -> Motor Input ring 2.3/1
  Dead Zone4/1 -> Motor Input ring 2.1/1
  Sine Wave Balala ring/1 -> Dead Zone1/1
  Sine Wave scissors ring/1 -> Dead Zone2/1
  Sine Wave swear ring/1 -> Dead Zone3/1

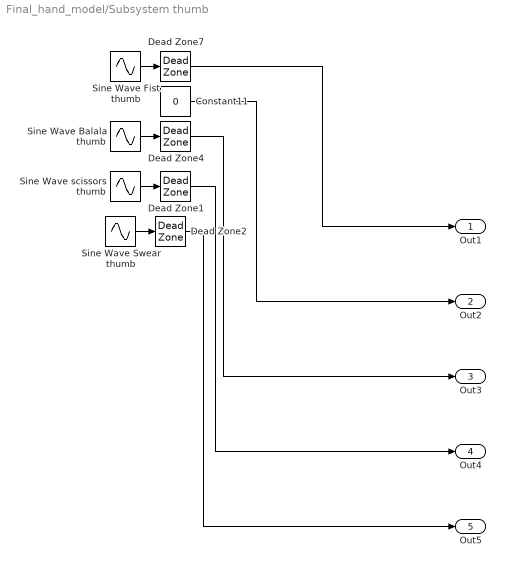
== system Final_hand_model/Subsystem thumb ==
  Constant11 : Constant  Value=0
  Dead Zone{1..2,4,7} (4 alike) : DeadZone  LowerValue=-10  UpperValue=0  SaturateOnIntegerOverflow=on
  Sine Wave Balala thumb : Sin  Amplitude=0.5  Frequency=3  Phase=4*pi/5  SampleTime=0
  Sine Wave Fist thumb : Sin  Amplitude=1.3  Frequency=3  SampleTime=0
  Sine Wave Swear thumb : Sin  Amplitude=1.3  Frequency=3  SampleTime=0
  Sine Wave scissors thumb : Sin  Amplitude=1.3  Frequency=3  SampleTime=0
  Out1 : Outport
  Out2 : Outport  Port=2
  Out3 : Outport  Port=3
  Out4 : Outport  Port=4
  Out5 : Outport  Port=5
  wires:
  Sine Wave Fist thumb/1 -> Dead Zone7/1
  Constant11/1 -> Out2/1
  Dead Zone7/1 -> Out1/1
  Dead Zone4/1 -> Out3/1
  Dead Zone2/1 -> Out5/1
  Sine Wave Swear thumb/1 -> Dead Zone2/1
  Sine Wave Balala thumb/1 -> Dead Zone4/1
  Sine Wave scissors thumb/1 -> Dead Zone1/1
  Dead Zone1/1 -> Out4/1

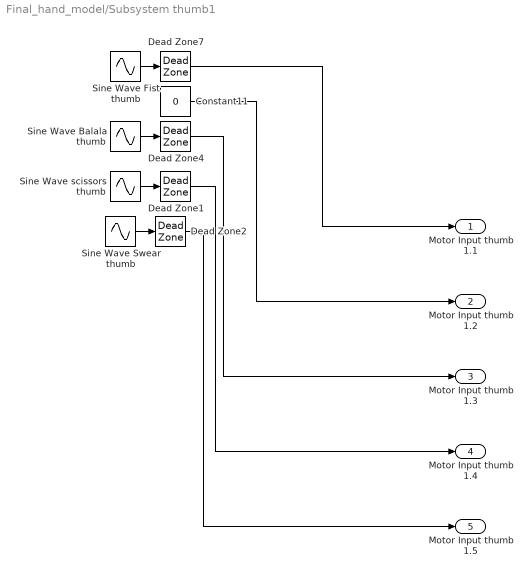
== system Final_hand_model/Subsystem thumb1 ==
  Constant11 : Constant  Value=0
  Dead Zone{1..2,4,7} (4 alike) : DeadZone  LowerValue=-10  UpperValue=0  SaturateOnIntegerOverflow=on
  Sine Wave Balala thumb : Sin  Amplitude=0.5  Frequency=3  Phase=4*pi/5  SampleTime=0
  Sine Wave Fist thumb : Sin  Amplitude=1.3  Frequency=3  SampleTime=0
  Sine Wave Swear thumb : Sin  Amplitude=1.3  Frequency=3  SampleTime=0
  Sine Wave scissors thumb : Sin  Amplitude=1.3  Frequency=3  SampleTime=0
  Motor Input thumb 1.1 : Outport
  Motor Input thumb 1.2 : Outport  Port=2
  Motor Input thumb 1.3 : Outport  Port=3
  Motor Input thumb 1.4 : Outport  Port=4
  Motor Input thumb 1.5 : Outport  Port=5
  wires:
  Sine Wave Fist thumb/1 -> Dead Zone7/1
  Constant11/1 -> Motor Input thumb 1.2/1
  Dead Zone7/1 -> Motor Input thumb 1.1/1
  Dead Zone4/1 -> Motor Input thumb 1.3/1
  Dead Zone2/1 -> Motor Input thumb 1.5/1
  Sine Wave Swear thumb/1 -> Dead Zone2/1
  Sine Wave Balala thumb/1 -> Dead Zone4/1
  Sine Wave scissors thumb/1 -> Dead Zone1/1
  Dead Zone1/1 -> Motor Input thumb 1.4/1

== system Final_hand_model/Subsystem wrist ==
  Balala : Constant  Value=0
  Fist : Constant  Value=0
  Sine Wave Openhand wrist : Sin  Amplitude=0.5  Frequency=3  SampleTime=0
  scissors : Constant  Value=0
  swear : Constant  Value=0
  Out1 : Outport
  Out2 : Outport  Port=2
  Out3 : Outport  Port=3
  Out4 : Outport  Port=4
  Out5 : Outport  Port=5
  wires:
  Balala/1 -> Out3/1
  Sine Wave Openhand wrist/1 -> Out2/1
  Fist/1 -> Out1/1
  swear/1 -> Out5/1
  scissors/1 -> Out4/1

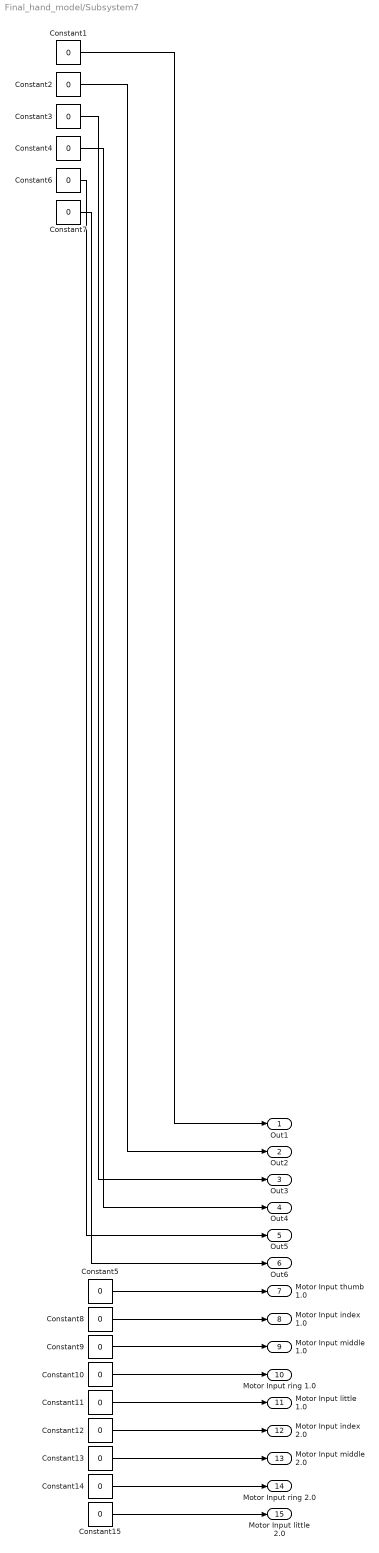
== system Final_hand_model/Subsystem7 ==
  Constant{1..15} (15 alike) : Constant  Value=0
  Out1 : Outport
  Out2 : Outport  Port=2
  Out3 : Outport  Port=3
  Out4 : Outport  Port=4
  Out5 : Outport  Port=5
  Out6 : Outport  Port=6
  Motor Input thumb 1.0 : Outport  Port=7
  Motor Input index 1.0 : Outport  Port=8
  Motor Input middle 1.0 : Outport  Port=9
  Motor Input ring 1.0 : Outport  Port=10
  Motor Input little 1.0 : Outport  Port=11
  Motor Input index 2.0 : Outport  Port=12
  Motor Input middle 2.0 : Outport  Port=13
  Motor Input ring 2.0 : Outport  Port=14
  Motor Input little 2.0 : Outport  Port=15
  wires:
  Constant3/1 -> Out3/1
  Constant6/1 -> Out5/1
  Constant1/1 -> Out1/1
  Constant2/1 -> Out2/1
  Constant4/1 -> Out4/1
  Constant7/1 -> Out6/1
  Constant15/1 -> Motor Input little 2.0/1
  Constant14/1 -> Motor Input ring 2.0/1
  Constant13/1 -> Motor Input middle 2.0/1
  Constant12/1 -> Motor Input index 2.0/1
  Constant11/1 -> Motor Input little 1.0/1
  Constant10/1 -> Motor Input ring 1.0/1
  Constant9/1 -> Motor Input middle 1.0/1
  Constant8/1 -> Motor Input index 1.0/1
  Constant5/1 -> Motor Input thumb 1.0/1
